simulink library "Lamp_Lib"  (R2014a)
settings: Solver=ode45  StartTime=0.0  StopTime=10.0  RelTol=1e-3
undefined symbols (not defined in the file): APN_Param
libraries: Lamp_Lib x3, powerlib x2
Description:
  | Copyright 2014 The MathWorks, Inc.
settings Model: Creator=smiller  LastModifiedBy=psanghvi

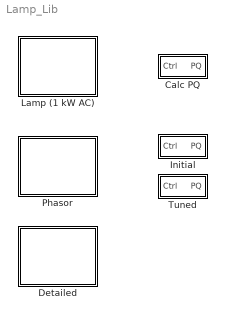
== system Lamp_Lib ==
  Calc PQ : Subsystem  BlockChoice=Initial
      settings: TemplateBlock=self  MemberBlocks=Initial,Tuned
  Detailed : Subsystem
      mask Display: image(imread('LampAC_Detailed_IMAGE.jpg'));
  Initial : Subsystem
  Lamp (1 kW AC) : Subsystem  BlockChoice=Detailed
      settings: TemplateBlock=self  MemberBlocks=Detailed,Phasor
  Phasor : Subsystem
      mask Display: image(imread('LampAC_Phasor_IMAGE.jpg'));
  Tuned : Subsystem

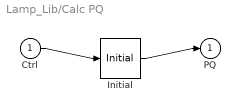
== system Lamp_Lib/Calc PQ ==
  Ctrl : Inport
  Initial : Lamp_Lib/Initial
  PQ : Outport
  wires:
  Ctrl/1 -> Initial/1
  Initial/1 -> PQ/1

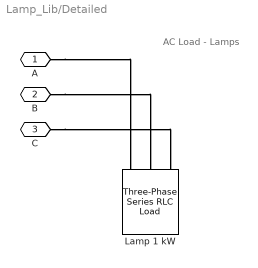
== system Lamp_Lib/Detailed ==
  note: AC Load - Lamps
  Lamp 1 kW : powerlib/Elements/Three-Phase Series RLC Load  LConnTagsString=A|B|C  Configuration=Y (grounded)  NominalVoltage=200  NominalFrequency=400  ActivePower=1000  InductivePower=0  CapacitivePower=0  Measurements=None  LoadType=constant Z
  A : PMIOPort  Port=1  Side=Left
  B : PMIOPort  Port=2  Side=Left
  C : PMIOPort  Port=3  Side=Left
  connections:
  A/RConn1 -- Lamp 1 kW/LConn1
  B/RConn1 -- Lamp 1 kW/LConn2
  C/RConn1 -- Lamp 1 kW/LConn3

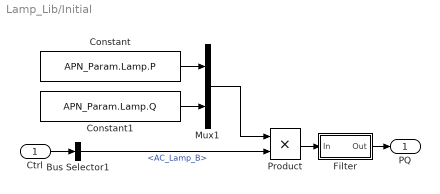
== system Lamp_Lib/Initial ==
  Ctrl : Inport
  Bus Selector1 : BusSelector  OutputSignals=AC_Lamp_B
  Constant : Constant  Value=APN_Param.Lamp.P
  Constant1 : Constant  Value=APN_Param.Lamp.Q
  Filter : Subsystem  mask(First-order lag supporting vector signals){b=1e-2, x_initial=[APN_Param.Lamp.P APN_Param.Lamp.Q]*0}
      mask prompts: b "Filter time constant"; x_initial "Initial output"
      mask help: Models a lag of the form 1/(b*s+1) where s is the Laplace operator.
  Mux1 : Mux  Inputs=2
  Product : Product
  PQ : Outport
  wires:
  Ctrl/1 -> Bus Selector1/1
  Bus Selector1/1 -> Product/2  "<AC_Lamp_B>"
  Filter/1(Out) -> PQ/1
  Mux1/1 -> Product/1
  Constant/1 -> Mux1/1
  Constant1/1 -> Mux1/2
  Product/1 -> Filter/1(In)

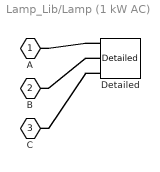
== system Lamp_Lib/Lamp (1 kW AC) ==
  Detailed : Lamp_Lib/Detailed  SystemSampleTime=-1
  A : PMIOPort  Port=1  Side=Left
  B : PMIOPort  Port=2  Side=Left
  C : PMIOPort  Port=3  Side=Left
  connections:
  Detailed/LConn1 -- A/RConn1
  Detailed/LConn2 -- B/RConn1
  Detailed/LConn3 -- C/RConn1

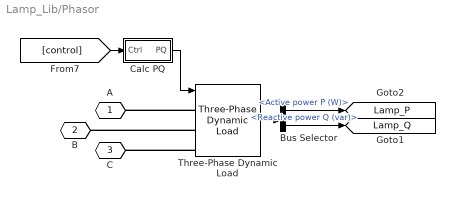
== system Lamp_Lib/Phasor ==
  Bus Selector : BusSelector  OutputSignals=Active power P (W),Reactive power Q (var)
  Calc PQ : Subsystem  BlockChoice=Initial
      settings: AttributesFormatString=%<BlockChoice>  TemplateBlock=Lamp_Lib/Calc PQ  MemberBlocks=Initial,Tuned
  Three-Phase Dynamic Load : powerlib/Elements/Three-Phase Dynamic Load  NominalVoltage=[ 200 400 ]  ActiveReactivePowers=[APN_Param.Lamp.P APN_Param.Lamp.Q]*0  PositiveSequence=[0.0004 0]  ExternalControl=on  NpNq=[1.3 2]  TimeConstants="[0  0  0  0]"  MinimumVoltage=0.7  LoadFlowParameters=[4 0 0 0 0]
  A : PMIOPort  Port=1  Side=Left
  B : PMIOPort  Port=2  Side=Left
  C : PMIOPort  Port=3  Side=Left
  tag scope: Lamp_P=global, Lamp_Q=global
  wires:
  Bus Selector/1 -> [Lamp_P]  "<Active power P (W)>"
  Three-Phase Dynamic Load/1 -> Bus Selector/1
  Bus Selector/2 -> [Lamp_Q]  "<Reactive power Q (var)>"
  [control] -> Calc PQ/1(Ctrl)
  Calc PQ/1(PQ) -> Three-Phase Dynamic Load/1
  connections:
  Three-Phase Dynamic Load/LConn3 -- C/RConn1
  Three-Phase Dynamic Load/LConn2 -- B/RConn1
  Three-Phase Dynamic Load/LConn1 -- A/RConn1

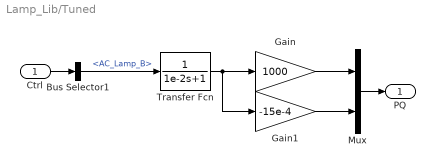
== system Lamp_Lib/Tuned ==
  Ctrl : Inport
  Bus Selector1 : BusSelector  OutputSignals=AC_Lamp_B
  Gain : Gain  Gain=1000
  Gain1 : Gain  Gain=-15e-4
  Mux : Mux  Inputs=2
  Transfer Fcn : TransferFcn  Denominator=[1e-2 1]
  PQ : Outport
  wires:
  Mux/1 -> PQ/1
  Transfer Fcn/1 -> Gain1/1, Gain/1
  Gain/1 -> Mux/1
  Gain1/1 -> Mux/2
  Bus Selector1/1 -> Transfer Fcn/1  "<AC_Lamp_B>"
  Ctrl/1 -> Bus Selector1/1

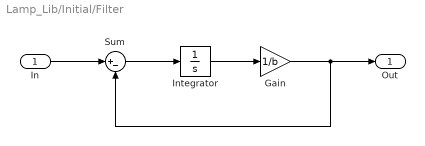
== system Lamp_Lib/Initial/Filter ==
  In : Inport
  Gain : Gain  Gain=1/b
  Integrator : Integrator  InitialCondition=x_initial
  Sum : Sum  Inputs=|+-  SaturateOnIntegerOverflow=on  InputSameDT=on  OutDataTypeStr=Inherit: Same as first input
  Out : Outport
  wires:
  Gain/1 -> Out/1, Sum/2
  Integrator/1 -> Gain/1
  In/1 -> Sum/1
  Sum/1 -> Integrator/1

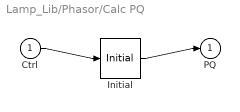
== system Lamp_Lib/Phasor/Calc PQ ==
  Ctrl : Inport
  Initial : Lamp_Lib/Initial
  PQ : Outport
  wires:
  Ctrl/1 -> Initial/1
  Initial/1 -> PQ/1
